simulink model "power_voltmeasure"  (Simulink 6.0)
settings: Solver=ode15s  SolverMode=SingleTasking  StartTime=0.0  StopTime=0.1  RelTol=1e-3  AbsTol=1e-6
libraries: powerlib x14
settings Model: Creator=patrice  LastModifiedBy=batserve  ExtModeTrigMode=oneshot  ExtModeArmWhenConnect=off  ExtModeAutoUpdateStatusClock=off
settings DataIOCC: LimitDataPoints=off  SignalLoggingName=sigsOut
settings OptimizationCC: BooleanDataType=off
settings DebuggingCC: SolverPrmCheckMsg=none
settings HardwareCC: TargetUnknown=on
settings RTWCC: TemplateMakefile=grt_unix.tmf

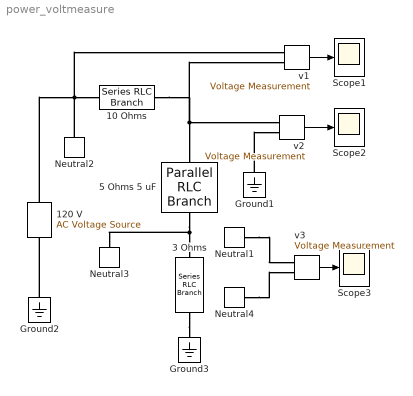
== system power_voltmeasure ==
  10 Ohms : powerlib/Elements/Series RLC Branch  PhysicalDomain=powersysdomain  SubClassName=unknown  PortType=p1  LConnTagsString=__new0  RConnTagsString=__new0  Resistance=10  Inductance=0  Capacitance=inf  Measurements=None
  120 V : powerlib/Electrical Sources/AC Voltage Source  Description=source block  Orientation=up  Amplitude=120  Phase=0  Frequency=60  SampleTime=0  Measurements=None
      settings: AttributesFormatString=\n
  3 Ohms : powerlib/Elements/Series RLC Branch  Orientation=down  PhysicalDomain=powersysdomain  SubClassName=unknown  PortType=p1  LConnTagsString=__new0  RConnTagsString=__new0  Resistance=3  Inductance=0  Capacitance=inf  Measurements=None
  5 Ohms 5 uF : powerlib/Elements/Parallel RLC Branch  Orientation=down  PhysicalDomain=powersysdomain  SubClassName=unknown  PortType=p1  LConnTagsString=a  RConnTagsString=__new0  Resistance=5  Inductance=inf  Capacitance=5e-6  Measurements=None
  Ground1 : powerlib/Elements/Ground  Orientation=down  PhysicalDomain=powersysdomain  SubClassName=unknown  PortType=p1  LConnTagsString=a
  Ground2 : powerlib/Elements/Ground  Orientation=down  PhysicalDomain=powersysdomain  SubClassName=unknown  PortType=p1  LConnTagsString=a
  Ground3 : powerlib/Elements/Ground  Orientation=down  PhysicalDomain=powersysdomain  SubClassName=unknown  PortType=p1  LConnTagsString=a
  Neutral1 : powerlib/Elements/Neutral  Orientation=left  PhysicalDomain=powersysdomain  SubClassName=unknown  PortType=p1  LConnTagsString=a  NodeNumber=10
  Neutral2 : powerlib/Elements/Neutral  Orientation=down  PhysicalDomain=powersysdomain  SubClassName=unknown  PortType=p1  LConnTagsString=a  NodeNumber=10
  Neutral3 : powerlib/Elements/Neutral  Orientation=down  PhysicalDomain=powersysdomain  SubClassName=unknown  PortType=p1  LConnTagsString=a  NodeNumber=20
  Neutral4 : powerlib/Elements/Neutral  Orientation=left  PhysicalDomain=powersysdomain  SubClassName=unknown  PortType=p1  LConnTagsString=a  NodeNumber=20
  Scope1 : Scope
      settings: TickLabels=on  TimeRange=0.1  YMin=-100  YMax=100  DataFormat=Array
  Scope2 : Scope
      settings: TickLabels=on  TimeRange=0.1  YMin=-60  YMax=60  DataFormat=Array
  Scope3 : Scope
      settings: TickLabels=on  TimeRange=0.1  YMin=-120  YMax=120  DataFormat=Array
  v1 : powerlib/Measurements/Voltage Measurement  Tag=PoWeRsYsTeMmEaSuReMeNt  PhasorSimulation=off  OutputType=Magnitude  PSBequivalent=0
  v2 : powerlib/Measurements/Voltage Measurement  Tag=PoWeRsYsTeMmEaSuReMeNt  PhasorSimulation=off  OutputType=Magnitude  PSBequivalent=0
  v3 : powerlib/Measurements/Voltage Measurement  Tag=PoWeRsYsTeMmEaSuReMeNt  PhasorSimulation=off  OutputType=Magnitude  PSBequivalent=0
  wires:
  v2/1 -> Scope2/1
  v1/1 -> Scope1/1
  v3/1 -> Scope3/1
  connections:
  Neutral1/LConn1 -- v3/LConn1
  Neutral4/LConn1 -- v3/LConn2
  Ground1/LConn1 -- v2/LConn2
  3 Ohms/RConn1 -- Ground3/LConn1
  5 Ohms 5 uF/RConn1 -- 3 Ohms/LConn1 -- Neutral3/LConn1
  10 Ohms/RConn1 -- v1/LConn2 -- 5 Ohms 5 uF/LConn1 -- v2/LConn1
  Neutral2/LConn1 -- 10 Ohms/LConn1 -- v1/LConn1 -- 120 V/RConn1
  Ground2/LConn1 -- 120 V/LConn1
